simulink model "Lab_2_Sim_5"  (R2023b)
settings: Solver=VariableStepAuto  StartTime=0.0  StopTime=20.0  RelTol=1e-3
values from neighbouring files (symbols this model uses):
  G_den = [M B k]    [Lab_2_Num1.m]    (also in Lab_2_Num2.m; Lab_2_Num3.m; Lab_2_Num5.m = [1 2 3 4 5 6 7 1]; Lab_2_Num6.m = [1 2 3 4 1])
  G_num = [1 ]    [Lab_2_Num1.m]    (also in Lab_2_Num2.m = [1]; Lab_2_Num3.m = [1]; Lab_2_Num5.m = [8 7 6 5 4 3 2]; Lab_2_Num6.m = [4 3 2 1])
settings Model: Creator=ACER 1  LastModifiedBy=Dell

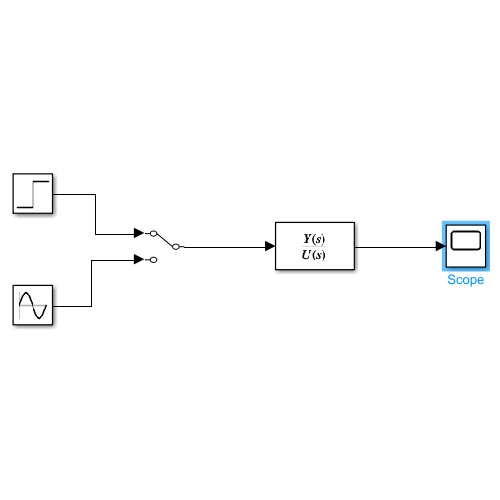
[thumbnail: Simulink's stored preview of the top-level diagram]
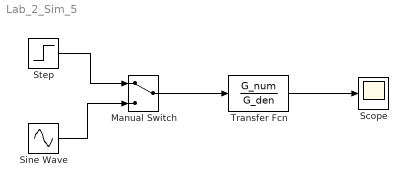
== system Lab_2_Sim_5 ==
  Manual Switch : ManualSwitch
  Scope : Scope
  Sine Wave : Sin  SampleTime=0
  Step : Step  Time=0  SampleTime=0
  Transfer Fcn : TransferFcn  Numerator=G_num  Denominator=G_den  ParameterTunability=Unconstrained
  wires:
  Manual Switch/1 -> Transfer Fcn/1
  Transfer Fcn/1 -> Scope/1
  Step/1 -> Manual Switch/1
  Sine Wave/1 -> Manual Switch/2
